simulink model "GVCU_HIL_simscape"  (R2026a)
settings: Solver=ode3  StartTime=0  StopTime=10  FixedStep=0.001
model workspace (MAT data in the model file):
  CANoelibParameters : object (value not decoded)
values from neighbouring files (symbols this model uses):
  acc_pedal_data = pedal_data.accelerator_pedal_position_t0    [Init_Simscape_main.m]
  acc_pedal_time = pedal_data.t0    [Init_Simscape_main.m]
  brk_pedal_data = brake_pedal_data.shared_brakes_drvrBrkPedlPerc_t0    [Init_Simscape_main.m]
  brk_pedal_time = brake_pedal_data.t0    [Init_Simscape_main.m]
  cycle_len = zeros(1, num_cycles)    [Init_Simscape_main.m]
  cycle_speed_matrix = zeros(max_cycle_len, num_cycles)    [Init_Simscape_main.m]
  cycle_time_matrix = zeros(max_cycle_len, num_cycles)    [Init_Simscape_main.m]
  veh_speed_data = speed_data.shared_dynamicsVso_vehVelLgt_t0    [Init_Simscape_main.m]
  veh_speed_time = speed_data.t0    [Init_Simscape_main.m]
undefined symbols (not defined in the file or in its folder): Active, aero, AuxActive, bat, brake, config, environment, FL, FL_prs_voltage, FR, FR_prs_voltage, front, pos, powertrain, rear, RL, RL_prs_voltage, RR, RR_prs_voltage, tir, veh, VGetRawValueFlag, Voltage, VT2816_1_Ch1, VT2816_1_Ch2, VT2816_1_Ch3, VT2816_1_Ch4, VT2816_3_Ch13, VT2816_3_Ch14, VT7101_1_Out2, VTS, X, Y, Z
libraries: sm_lib x358, fl_lib x272, nesl_utility x193, canoelib x127, sdl_lib x36, autolibsharedcoupling x21, autolibcoupling x9, slpidlib x7, simulink x3, autolibshareddiff x3, autolibshared x3, autolibutils x1
(part 7 of 17)

== system GVCU_HIL_simscape/Vehicle/to grade ==
  In1 : Inport
  Constant : Constant  Value=veh.f + veh.r
  Divide : Product  Inputs=*/
  Gain : Gain  Gain=0.5
  Gain1 : Gain  Gain=0.5
  "Radians to Degrees " : simulink_extras/Transformations/Radians to Degrees
  Selector : Selector  InputPortWidth=4  IndexOptions=Index vector (dialog)  Indices=[1]  OutputSizes=1
  Selector1 : Selector  InputPortWidth=4  IndexOptions=Index vector (dialog)  Indices=[2]  OutputSizes=1
  Selector2 : Selector  InputPortWidth=4  IndexOptions=Index vector (dialog)  Indices=[3]  OutputSizes=1
  Selector3 : Selector  InputPortWidth=4  IndexOptions=Index vector (dialog)  Indices=[4]  OutputSizes=1
  Sum : Sum
  Sum1 : Sum
  Sum2 : Sum  Inputs=+-
  "Tan " : Trigonometry  Operator=asin
  Out1 : Outport
  wires:
  "Radians to Degrees "/1 -> Out1/1
  "Tan "/1 -> "Radians to Degrees "/1
  Divide/1 -> "Tan "/1
  Constant/1 -> Divide/2
  Sum2/1 -> Divide/1
  Gain1/1 -> Sum2/2
  Gain/1 -> Sum2/1
  Sum1/1 -> Gain1/1
  Sum/1 -> Gain/1
  Selector3/1 -> Sum1/2
  Selector2/1 -> Sum1/1
  Selector1/1 -> Sum/2
  Selector/1 -> Sum/1
  In1/1 -> Selector/1, Selector1/1, Selector2/1, Selector3/1
